simulink model "EZE4sFlow"  (R2018b)
settings: Solver=FixedStepDiscrete  StartTime=0.0  StopTime=10.0  FixedStep=0.01  RelTol=1e-3
settings Model: ModifiedHistory=2023.8.1 V2.0.0 CR421790 增加模式21-26  Creator=sn2xws  LastModifiedBy=sn2xws
settings DataIOCC: SaveFormat=StructureWithTime
settings OptimizationCC: DefaultParameterBehavior=Inlined  EnhancedBackFolding=on  PassReuseOutputArgsAs=Individual arguments  ZeroExternalMemoryAtStartup=off  ZeroInternalMemoryAtStartup=off  OptimizeBlockOrder=speed  DifferentSizesBufferReuse=on  OptimizationCustomize=off
settings DebuggingCC: ParameterTunabilityLossMsg=error
settings SFSimCC: MATLABDynamicMemAlloc=off
settings RTWCC: SystemTargetFile=autosar.tlc  GenCodeOnly=on  TemplateMakefile=ert_default_tmf  Description=AUTOSAR  GenerateReport=on  IncludeHyperlinkInReport=on  LaunchReport=on  GenerateTraceInfo=on  GenerateTraceReport=on  GenerateTraceReportSl=on  GenerateTraceReportSf=on  GenerateTraceReportEml=on  GenerateCodeMetricsReport=on
settings CodeAppCC: ForceParamTrailComments=on  IgnoreCustomStorageClasses=off  OperatorAnnotations=on  SimulinkDataObjDesc=on  SFDataObjDesc=on  InsertBlockDesc=on
settings STFCustomTargetCC: TargetLangStandard=C99 (ISO)  MultiwordLength=256  ParMdlRefBuildCompliant=on  CompOptLevelCompliant=on  IncludeMdlTerminateFcn=off  CombineOutputUpdateFcns=on  SuppressErrorStatus=on  ERTCustomFileBanners=on  SupportNonFinite=off  SupportComplex=off  SupportContinuousTime=off  SupportNonInlinedSFcns=off  RemoveResetFunc=on  MATLABClassNameForMDSCustomization=Simulink.SoftwareTarget.ERTCustomization  AutosarCompliant=on  UseToolchainInfoCompliant=on  LookupTableObjectStructAxisOrder=2,1,3,4,...  LUTObjectStructOrderEvenSpacing=Size,Table,Breakpoints  SystemTargetFile=autosar.tlc
settings ERTTargetCC: TargetLangStandard=C99 (ISO)  ConcurrentExecutionCompliant=off  IncludeMdlTerminateFcn=off  SuppressErrorStatus=on  SupportNonFinite=off  SupportComplex=off  ModelStepFunctionPrototypeControlCompliant=off  CPPClassGenCompliant=off  AutosarCompliant=on  LookupTableObjectStructAxisOrder=2,1,3,4,...  LUTObjectStructOrderEvenSpacing=Size,Table,Breakpoints  InlinedParameterPlacement=NonHierarchical  ERTCustomFileTemplate=example_file_process.tlc  ERTFilePackagingFormat=Compact

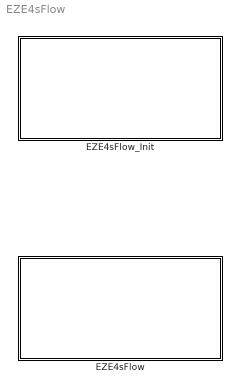
== system EZE4sFlow ==
  EZE4sFlow : Subsystem
  EZE4sFlow_Init : Subsystem

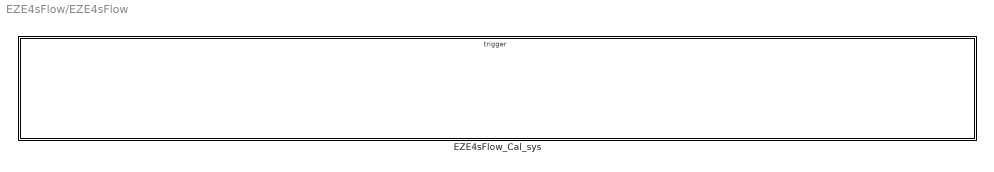
== system EZE4sFlow/EZE4sFlow ==
  EZE4sFlow_Cal_sys : Subsystem

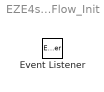
== system EZE4sFlow/EZE4sFlow_Init ==
  Event Listener : EventListener  EventName=reset

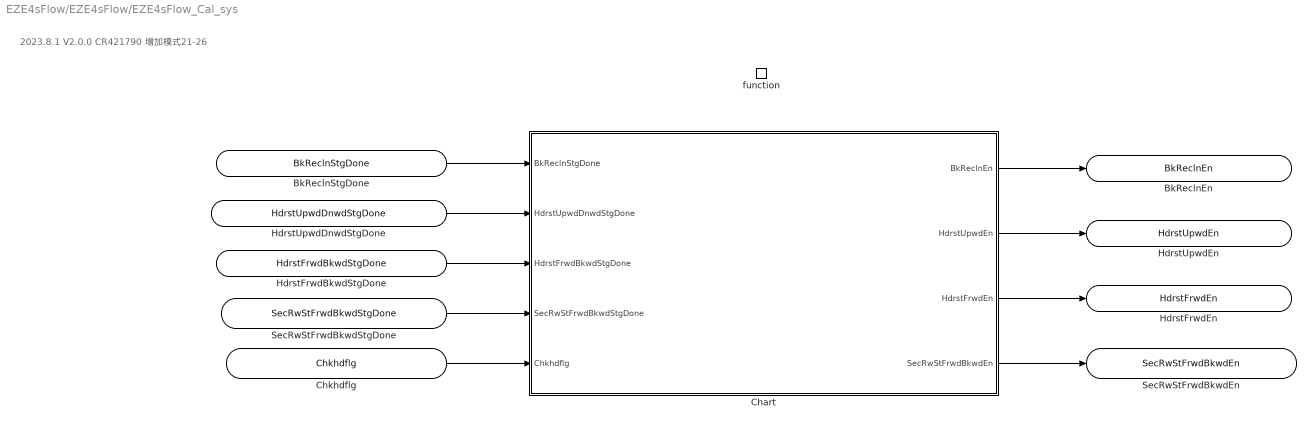
== system EZE4sFlow/EZE4sFlow/EZE4sFlow_Cal_sys ==
  note: 2023.8.1 V2.0.0 CR421790 增加模式21-26
  function : TriggerPort  TriggerType=function-call  IsSimulinkFunction=on  FunctionName=EZE4sFlow_Cal  VariantControl=(inherit)
  Chart : Stateflow chart  TreatAsAtomicUnit=on
  BkReclnStgDone : ArgIn  OutDataTypeStr=boolean  ArgumentName=BkReclnStgDone
  HdrstUpwdDnwdStgDone : ArgIn  Port=2  OutDataTypeStr=boolean  ArgumentName=HdrstUpwdDnwdStgDone
  HdrstFrwdBkwdStgDone : ArgIn  Port=3  OutDataTypeStr=boolean  ArgumentName=HdrstFrwdBkwdStgDone
  SecRwStFrwdBkwdStgDone : ArgIn  Port=4  OutDataTypeStr=boolean  ArgumentName=SecRwStFrwdBkwdStgDone
  Chkhdflg : ArgIn  Port=5  OutDataTypeStr=boolean  ArgumentName=Chkhdflg
  BkReclnEn : ArgOut  OutDataTypeStr=boolean  ArgumentName=BkReclnEn
  HdrstUpwdEn : ArgOut  Port=2  OutDataTypeStr=boolean  ArgumentName=HdrstUpwdEn
  HdrstFrwdEn : ArgOut  Port=3  OutDataTypeStr=boolean  ArgumentName=HdrstFrwdEn
  SecRwStFrwdBkwdEn : ArgOut  Port=4  OutDataTypeStr=boolean  ArgumentName=SecRwStFrwdBkwdEn
  wires:
  BkReclnStgDone/1 -> Chart/1(BkReclnStgDone)
  HdrstUpwdDnwdStgDone/1 -> Chart/2(HdrstUpwdDnwdStgDone)
  HdrstFrwdBkwdStgDone/1 -> Chart/3(HdrstFrwdBkwdStgDone)
  SecRwStFrwdBkwdStgDone/1 -> Chart/4(SecRwStFrwdBkwdStgDone)
  Chkhdflg/1 -> Chart/5(Chkhdflg)
  Chart/4(SecRwStFrwdBkwdEn) -> SecRwStFrwdBkwdEn/1
  Chart/3(HdrstFrwdEn) -> HdrstFrwdEn/1
  Chart/1(BkReclnEn) -> BkReclnEn/1
  Chart/2(HdrstUpwdEn) -> HdrstUpwdEn/1

== stateflow chart EZE4sFlow/EZE4sFlow_Cal_sys/Chart ==
  (default) -> (junction 10) : {
      | BkReclnEn = 0;
      | HdrstUpwdEn=0;
      | HdrstFrwdEn = 0;
      | SecRwStFrwdBkwdEn = 0;
      | }
  (junction 10) -> (junction 12) [order 1] : [BkReclnStgDone]
  (junction 10) -> (junction 14) [order 2] : {BkReclnEn=1;}
  (junction 12) -> (junction 16)
  (junction 16) -> (junction 14)
  (junction 14) -> (junction 19)
  (junction 19) -> (junction 21) [order 1] : [SecRwStFrwdBkwdStgDone]
  (junction 19) -> (junction 25) [order 2] : {SecRwStFrwdBkwdEn = 1;}
  (junction 21) -> (junction 23)
  (junction 23) -> (junction 25)
  (junction 25) -> (junction 50)
  (junction 50) -> (junction 45) [order 1] : [Chkhdflg]
  (junction 45) -> (junction 46) [order 1] : [HdrstUpwdDnwdStgDone]
  (junction 46) -> (junction 47) [order 1] : [HdrstFrwdBkwdStgDone]
  (junction 50) -> (junction 48) [order 2]
  (junction 45) -> (junction 57) [order 2] : {
      | HdrstUpwdEn=1;
      | }
  (junction 46) -> (junction 59) [order 2] : {
      | HdrstFrwdEn=1;
      | }
  (junction 47) -> (junction 60)
  (junction 48) -> (junction 49) [order 1] : [HdrstUpwdDnwdStgDone]
  (junction 48) -> (junction 51) [order 2] : {
      | HdrstUpwdEn=1;
      | }
  (junction 49) -> (junction 52)
  (junction 52) -> (junction 51)
  (junction 51) -> (junction 53)
  (junction 53) -> (junction 55) [order 1] : [HdrstFrwdBkwdStgDone]
  (junction 53) -> (junction 54) [order 2] : {
      | HdrstFrwdEn=1;
      | }
  (junction 55) -> (junction 58)
  (junction 58) -> (junction 54)
  (junction 54) -> (junction 56)
  (junction 57) -> (junction 56)
  (junction 59) -> (junction 57)
  (junction 60) -> (junction 59)
  (junction 56) -> (junction 68)
  data: BkReclnStgDone input; HdrstUpwdDnwdStgDone input; HdrstFrwdBkwdStgDone input; SecRwStFrwdBkwdStgDone input; Chkhdflg input; BkReclnEn output; HdrstUpwdEn output; HdrstFrwdEn output; SecRwStFrwdBkwdEn output
